simulink model "mconversion_enumDT"  (Simulink 7.2)
settings: Solver=ode3  StartTime=0.0  StopTime=20  FixedStep=0.01  RelTol=1e-3
PreLoadFcn:
  | e1 = Simulink.BusElement;
  | e1.Name = 'foo_1';
  | e1.DataType = '?dEnumDT';
  | e2 = Simulink.BusElement;
  | e2.Name = 'foo_2';
  | e2.DataType = '?dEnumDT';
  | EnumType_Bus = Simulink.Bus;
  | EnumType_Bus.Elements = [e1 e2];
  | 
  | % Work around bug in MCOS.
  | BogusVar = dEnumDT.a;
settings Model: Creator=mwilkins  LastModifiedBy=mwilkins
settings DataIOCC: SaveOutput=off  SaveTime=off
settings OptimizationCC: InlineParams=on  InitFltsAndDblsToZero=on  EfficientMapNaN2IntZero=off
settings DebuggingCC: StrictBusMsg=ErrorLevel1

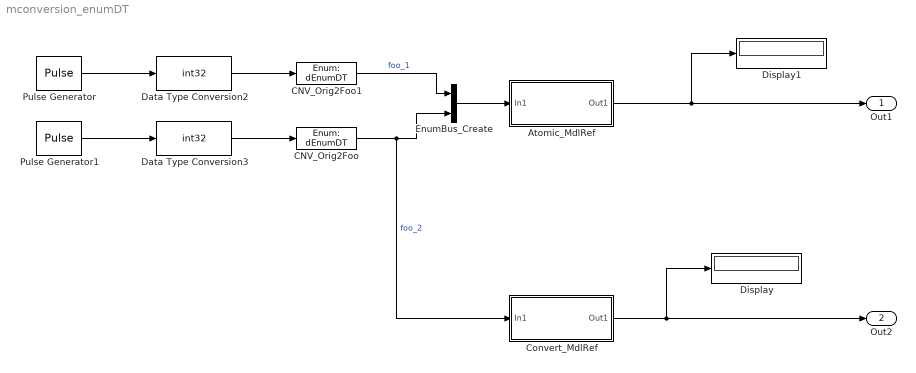
== system mconversion_enumDT ==
  Atomic_MdlRef : Subsystem  TreatAsAtomicUnit=on
  CNV_Orig2Foo : DataTypeConversion  OutDataTypeMode=Specify via dialog  OutDataType=Enum: dEnumDT  OutDataTypeStr=Enum: dEnumDT
  CNV_Orig2Foo1 : DataTypeConversion  OutDataTypeMode=Specify via dialog  OutDataType=Enum: dEnumDT  OutDataTypeStr=Enum: dEnumDT
  Convert_MdlRef : Subsystem  TreatAsAtomicUnit=on
  Data Type Conversion2 : DataTypeConversion  OutDataTypeMode=int32  OutDataType=sfix(16)  OutScaling=2^0  OutDataTypeStr=int32
  Data Type Conversion3 : DataTypeConversion  OutDataTypeMode=int32  OutDataType=sfix(16)  OutScaling=2^0  OutDataTypeStr=int32
  Display : Display
  Display1 : Display
  EnumBus_Create : BusCreator  Inputs=2  UseBusObject=on
      settings: BusObject=EnumType_Bus
  Pulse Generator : DiscretePulseGenerator  PulseType=Time based  PulseWidth=50
  Pulse Generator1 : DiscretePulseGenerator  PulseType=Time based  Amplitude=2  Period=5  PulseWidth=50
  Out1 : Outport  OutDataType=sfix(16)  OutScaling=2^0
  Out2 : Outport  Port=2  OutDataType=sfix(16)  OutScaling=2^0
  wires:
  EnumBus_Create/1 -> Atomic_MdlRef/1(In1)
  Atomic_MdlRef/1(Out1) -> Out1/1, Display1/1
  Pulse Generator/1 -> Data Type Conversion2/1
  Pulse Generator1/1 -> Data Type Conversion3/1
  CNV_Orig2Foo1/1 -> EnumBus_Create/1  "foo_1"
  Data Type Conversion2/1 -> CNV_Orig2Foo1/1
  Data Type Conversion3/1 -> CNV_Orig2Foo/1
  CNV_Orig2Foo/1 -> EnumBus_Create/2, Convert_MdlRef/1(In1)  "foo_2"
  Convert_MdlRef/1(Out1) -> Out2/1, Display/1

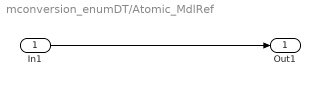
== system mconversion_enumDT/Atomic_MdlRef ==
  In1 : Inport  OutDataType=sfix(16)  OutScaling=2^0
  Out1 : Outport  OutDataType=sfix(16)  OutScaling=2^0
  wires:
  In1/1 -> Out1/1

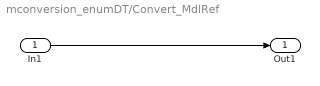
== system mconversion_enumDT/Convert_MdlRef ==
  In1 : Inport  OutDataType=sfix(16)  OutScaling=2^0
  Out1 : Outport  OutDataType=sfix(16)  OutScaling=2^0
  wires:
  In1/1 -> Out1/1
